simulink model "Test_TCPSocket_Client"  (Simulink 7.2)
settings: Solver=FixedStepDiscrete  StartTime=0.0  StopTime=10  RelTol=1e-6  AbsTol=1e-6
InitFcn:
  | clear('all');
settings Model: Creator=Andreas Schellenberg  LastModifiedBy=Andreas
settings DataIOCC: LimitDataPoints=off  SaveFormat=StructureWithTime  SaveState=on  SignalLogging=off  SignalLoggingName=sigsOut  OutputOption=SpecifiedOutputTimes  OutputTimes=t
settings OptimizationCC: InitFltsAndDblsToZero=on
settings DebuggingCC: SaveWithParameterizedLinksMsg=none  SignalResolutionControl=TryResolveAllWithWarning  SolverPrmCheckMsg=none  MultiTaskDSMMsg=warning  MultiTaskCondExecSysMsg=none  StrictBusMsg=None
settings HardwareCC: TargetUnknown=on
settings RTWCC: IncludeERTFirstTime=on

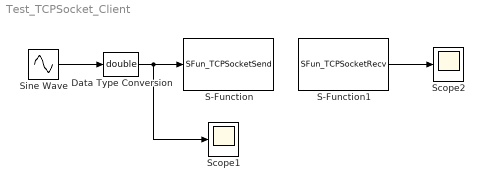
== system Test_TCPSocket_Client ==
  Data Type Conversion : DataTypeConversion  OutDataTypeMode=double  OutDataType=sfix(16)  OutScaling=2^0  OutDataTypeStr=double
  S-Function : S-Function  FunctionName=SFun_TCPSocketSend  Parameters=ipAddr,ipPort  EnableBusSupport=off  mask(TCPSocket Send){ipAddr=127.0.0.1, ipPort=8090}
      mask prompts: ipAddr "IP Address of Server (leave empty if defining a Server)"; ipPort "IP Port Number of Server or Client"
      mask Display: disp('TCPSocket\nSend');
  S-Function1 : S-Function  FunctionName=SFun_TCPSocketRecv  Parameters=ipAddr,ipPort,dataType,sampleTime  EnableBusSupport=off  mask(TCPSocket Receive){ipAddr=127.0.0.1, ipPort=8091, dataType=double, sampleTime=0.01}
      mask prompts: ipAddr "IP Address of Server (leave empty if defining a Server)"; ipPort "IP Port Number of Server or Client"; dataType "Data Type"; sampleTime "Sample Time"
      mask StyleString: edit,edit,popup(double|single|int32|int16|int8),edit
      mask Display: disp('TCPSocket\nReceive');
  Scope1 : Scope
      settings: TimeRange=10  YMin=-15  YMax=15
  Scope2 : Scope
      settings: TimeRange=10  YMin=-30  YMax=30
  Sine Wave : Sin  Amplitude=10  Frequency=pi  SampleTime=0.01
  wires:
  Sine Wave/1 -> Data Type Conversion/1
  S-Function1/1 -> Scope2/1
  Data Type Conversion/1 -> S-Function/1, Scope1/1
